simulink model "PVTOL_SMC_Asintotico"  (R2026b)
settings Model: Creator=nestorhernandezcastellanos  LastModifiedBy=nestorhernandezcastellanos

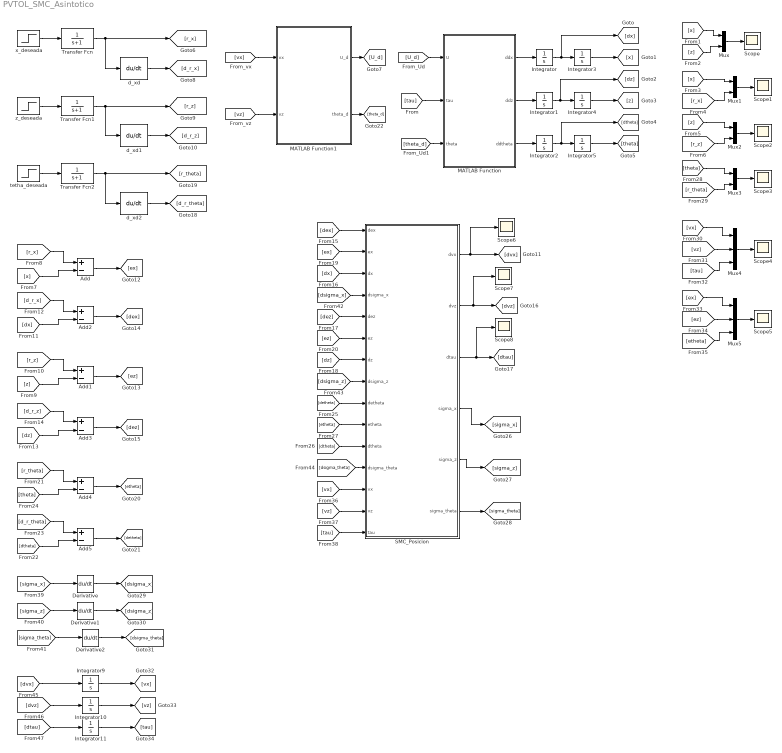
== system PVTOL_SMC_Asintotico ==
  Add{,1..5} (6 alike) : Sum  Inputs=+-
  Derivative : Derivative
  Derivative1 : Derivative
  Derivative2 : Derivative
  Integrator : Integrator  InitialCondition=2
  Integrator{1..2,4..5} (4 alike) : Integrator  InitialCondition=3
  Integrator10 : Integrator
  Integrator11 : Integrator
  Integrator3 : Integrator  InitialCondition=2
  Integrator9 : Integrator
  MATLAB Function : MATLAB Function  TreatAsAtomicUnit=on
  MATLAB Function1 : MATLAB Function  TreatAsAtomicUnit=on
  Mux{,1..3} (4 alike) : Mux  Inputs=2
  Mux4 : Mux  Inputs=3
  Mux5 : Mux  Inputs=3
  SMC_Posicion : MATLAB Function  TreatAsAtomicUnit=on
  Scope{,1..8} (9 alike) : Scope
      Scope settings: ActiveDisplayYMinimum=1.7015017403321495  ActiveDisplayYMaximum=4.686484337010655
      Scope1 settings: ActiveDisplayYMinimum=-0.62499999649831228  ActiveDisplayYMaximum=5.6249999684848113
      Scope2 settings: ActiveDisplayYMinimum=-0.62499999649831228  ActiveDisplayYMaximum=5.6249999684848113  DataLoggingVariableName=ScopeData2
      Scope3 settings: ActiveDisplayYMinimum=-0.62499999649831228  ActiveDisplayYMaximum=5.6249999684848113  DataLoggingVariableName=ScopeData3
      Scope4 settings: ActiveDisplayYMinimum=-6.5541537612794585  ActiveDisplayYMaximum=2.7221982614623772  DataLoggingVariableName=ScopeData4
      Scope5 settings: ActiveDisplayYMinimum=-5.0918407704159812  ActiveDisplayYMaximum=0.78910051784219049  DataLoggingVariableName=ScopeData5
      Scope6 settings: ActiveDisplayYMinimum=-375.96530288775057  ActiveDisplayYMaximum=375.89482808407041  DataLoggingVariableName=ScopeData6
      Scope7 settings: ActiveDisplayYMinimum=-375.96530288775057  ActiveDisplayYMaximum=375.89482808407041  DataLoggingVariableName=ScopeData7
      Scope8 settings: ActiveDisplayYMinimum=-375.96530288775057  ActiveDisplayYMaximum=375.89482808407041  DataLoggingVariableName=ScopeData8
  Transfer Fcn : TransferFcn  Denominator=[1 1]
  Transfer Fcn1 : TransferFcn  Denominator=[1 1]
  Transfer Fcn2 : TransferFcn  Denominator=[1 1]
  d_xd : Derivative
  d_xd1 : Derivative
  d_xd2 : Derivative
  tetha_deseada : Step  FinalValue=5  SampleTime=0
  x_deseada : Step  FinalValue=5  SampleTime=0
  z_deseada : Step  FinalValue=5  SampleTime=0
  wires:
  MATLAB Function/1(ddx) -> Integrator/1
  MATLAB Function/2(ddz) -> Integrator1/1
  MATLAB Function/3(ddtheta) -> Integrator2/1
  Integrator2/1 -> [dtheta], Integrator5/1
  Integrator1/1 -> [dz], Integrator4/1
  Integrator/1 -> [dx], Integrator3/1
  Integrator3/1 -> [x]
  Integrator4/1 -> [z]
  Integrator5/1 -> [theta]
  Mux/1 -> Scope/1
  [z] -> Mux/2
  [x] -> Mux/1
  x_deseada/1 -> Transfer Fcn/1
  Transfer Fcn/1 -> [r_x], d_xd/1
  [vx] -> MATLAB Function1/1(vx)
  [vz] -> MATLAB Function1/2(vz)
  [U_d] -> MATLAB Function/1(U)
  MATLAB Function1/1(U_d) -> [U_d]
  [x] -> Mux1/1
  [r_x] -> Mux1/2
  Mux1/1 -> Scope1/1
  Mux2/1 -> Scope2/1
  [r_z] -> Mux2/2
  [z] -> Mux2/1
  d_xd/1 -> [d_r_x]
  d_xd1/1 -> [d_r_z]
  Transfer Fcn1/1 -> d_xd1/1, [r_z]
  z_deseada/1 -> Transfer Fcn1/1
  [tau] -> MATLAB Function/2(tau)
  [r_x] -> Add/1
  [x] -> Add/2
  Add/1 -> [ex]
  [z] -> Add1/2
  [r_z] -> Add1/1
  Add2/1 -> [dex]
  [dx] -> Add2/2
  [d_r_x] -> Add2/1
  [d_r_z] -> Add3/1
  [dz] -> Add3/2
  Add3/1 -> [dez]
  SMC_Posicion/1(dvx) -> Scope6/1, [dvx]
  SMC_Posicion/2(dvz) -> Scope7/1, [dvz]
  SMC_Posicion/3(dtau) -> Scope8/1, [dtau]
  [dex] -> SMC_Posicion/1(dex)
  [dx] -> SMC_Posicion/3(dx)
  [dez] -> SMC_Posicion/5(dez)
  [dz] -> SMC_Posicion/7(dz)
  [ex] -> SMC_Posicion/2(ex)
  [ez] -> SMC_Posicion/6(ez)
  tetha_deseada/1 -> Transfer Fcn2/1
  Transfer Fcn2/1 -> [r_theta], d_xd2/1
  d_xd2/1 -> [d_r_theta]
  Add5/1 -> [detheta]
  [dtheta] -> Add5/2
  [d_r_theta] -> Add5/1
  [r_theta] -> Add4/1
  [theta] -> Add4/2
  [detheta] -> SMC_Posicion/9(detheta)
  [etheta] -> SMC_Posicion/10(etheta)
  [dtheta] -> SMC_Posicion/11(dtheta)
  MATLAB Function1/2(theta_d) -> [theta_d]
  [theta_d] -> MATLAB Function/3(theta)
  [theta] -> Mux3/1
  [r_theta] -> Mux3/2
  Mux3/1 -> Scope3/1
  Mux4/1 -> Scope4/1
  [vz] -> Mux4/2
  [vx] -> Mux4/1
  [tau] -> Mux4/3
  [etheta] -> Mux5/3
  [ex] -> Mux5/1
  [ez] -> Mux5/2
  Mux5/1 -> Scope5/1
  Add1/1 -> [ez]
  Add4/1 -> [etheta]
  SMC_Posicion/4(sigma_x) -> [sigma_x]
  SMC_Posicion/5(sigma_z) -> [sigma_z]
  SMC_Posicion/6(sigma_theta) -> [sigma_theta]
  [sigma_x] -> Derivative/1
  [sigma_z] -> Derivative1/1
  Derivative/1 -> [dsigma_x]
  Derivative1/1 -> [dsigma_z]
  Derivative2/1 -> [dsigma_theta]
  [sigma_theta] -> Derivative2/1
  [dsigma_x] -> SMC_Posicion/4(dsigma_x)
  [dsigma_z] -> SMC_Posicion/8(dsigma_z)
  [dsigma_theta] -> SMC_Posicion/12(dsigma_theta)
  [dvx] -> Integrator9/1
  [dvz] -> Integrator10/1
  [dtau] -> Integrator11/1
  Integrator9/1 -> [vx]
  Integrator10/1 -> [vz]
  Integrator11/1 -> [tau]
  [vx] -> SMC_Posicion/13(vx)
  [vz] -> SMC_Posicion/14(vz)
  [tau] -> SMC_Posicion/15(tau)

== matlab function PVTOL_SMC_Asintotico/MATLAB Function1 ==
  data: vx input; U_d output; vz input; theta_d output
function [U_d,theta_d] = linealizacion(vx,vz)

g = 9.81;                                  
U_d = sqrt(vx^2 + (vz+g)^2);                 
theta_d = atan2(-vx,vz+g);

== matlab function PVTOL_SMC_Asintotico/MATLAB Function ==
  data: U input; ddx output; tau input; theta input; ddz output; ddtheta output
function [ddx,ddz,ddtheta] = planta(U,tau,theta)

g = 9.81;                                       

ddx = -U*sin(theta);                            
ddz = U*cos(theta)-g;                           
ddtheta = tau;

== matlab function PVTOL_SMC_Asintotico/SMC_Posicion ==
  data: dex input; ex input; dx input; dsigma_x input; dez input; ez input; dz input; dsigma_z input; detheta input; etheta input; dtheta input; dsigma_theta input; vx input; dvx output; vz input; dvz output; dtau output; tau input; sigma_x output; sigma_z output; sigma_theta output
function [dvx, dvz, dtau, sigma_x, sigma_z, sigma_theta] = controlador(dex, ex, dx, dsigma_x, dez, ez, dz, dsigma_z, detheta, etheta, dtheta,dsigma_theta, vx, vz, tau)

% Parámetros del SMC asintótico
mx = 1;
mz = 1.8;
mtheta = 1.2;

msx = 30;
msz = 30;
mstheta = 25;

Kx = 40;
Kz = 40;
Ktheta = 25;

% Superficies principales
sigma_x = dex + mx*ex;
sigma_z = dez + mz*ez;
sigma_theta = detheta + mtheta*etheta;

% Superficies auxiliares
Sx = dsigma_x + msx*sigma_x;
Sz = dsigma_z + msz*sigma_z;
Stheta = dsigma_theta + mstheta*sigma_theta;

% Controladores dinámicos
dvx = -mx*msx*dx - (mx + msx)*vx + Kx*sign(Sx);
dvz = -mz*msz*dz - (mz + msz)*vz + Kz*sign(Sz);
dtau = -mtheta*mstheta*dtheta - (mtheta + mstheta)*tau + Ktheta*sign(Stheta);
